simulink library "cex_control_executive_lib"  (R2016b)
settings: Solver=ode45  StartTime=0.0  StopTime=10.0  RelTol=1e-3  EnableMultiTasking=on
undefined symbols (not defined in the file): ase_status_converged, ctl_idle_mode, ctl_stopped_mode, ctl_stopping_mode, ctl_stopping_omega_thresh, ctl_stopping_vel_thresh, tun_ctl_stopped_pos_thresh, tun_ctl_stopped_quat_thresh
libraries: simulink x7, cex_control_executive_lib x1, math_utils x1
settings Model: Creator=jfusco1  LastModifiedBy=jfusco1
settings DataIOCC: LimitDataPoints=on  SaveFormat=Array
settings OptimizationCC: LifeSpan=inf
settings DebuggingCC: AllowSymbolicDim=off  SFUnexpectedBacktrackingDiag=warning  SFNoUnconditionalDefaultTransitionDiag=warning  SFExecutionAtInitializationDiag=none
settings HardwareCC: ProdBitPerPointer=32  ProdBitPerSizeT=32  ProdBitPerPtrDiffT=32  ProdLargestAtomicFloat=None  ProdIntDivRoundTo=Undefined  ProdEndianess=Unspecified  ProdWordSize=32  ProdHWDeviceType=32-bit Generic
settings ModelReferenceCC: PropagateSignalLabelsOutOfModel=off
settings GRTTargetCC: TargetLangStandard=C89/C90 (ANSI)  GeneratePreprocessorConditionals=Disable all
settings ConfigComp: CovMetricSettings=dw  CovHtmlReporting=on  CovSaveCumulativeToWorkspaceVar=on  CovSaveSingleToWorkspaceVar=on  CovExternalEMLEnable=off

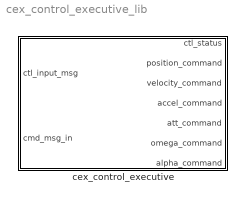
== system cex_control_executive_lib ==
  cex_control_executive : Subsystem

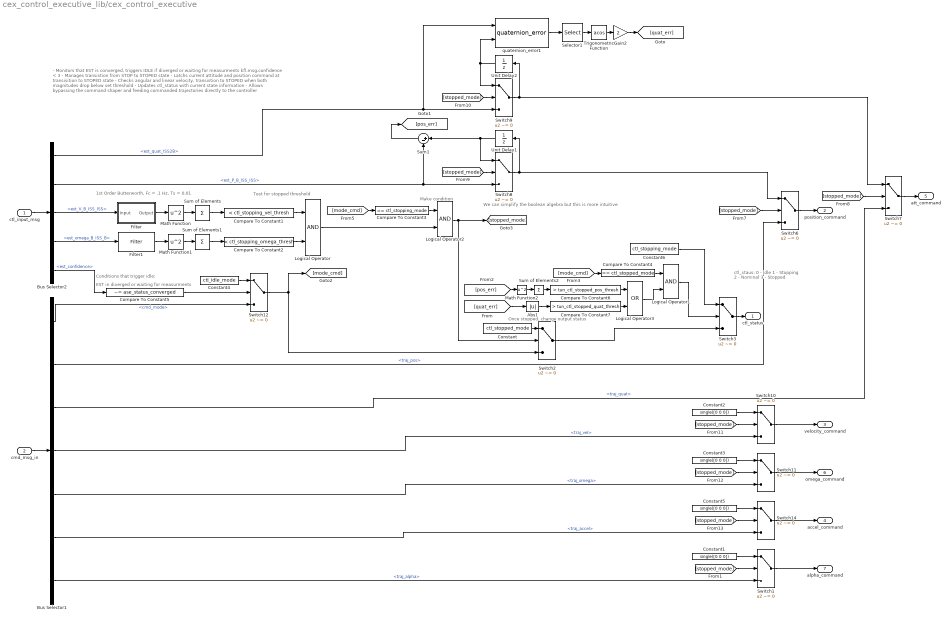
== system cex_control_executive_lib/cex_control_executive ==
  note: ctl_staus:
      | 0 - Idle
      | 1 - Stopping
      | 2 - Nominal
      | 3 - Stopped
  note: 1st Order Butterworth, Fc = .1 Hz, Ts = 0.01
  note: Once stopped, change output status
  note: Make condition
  note: We can simplify the boolean algebra but this is more intuitive
  note: Test for stopped threshold
  note: Conditions that trigger idle:
  note: EST in diverged or waiting for measurments
  note: - Monitors that EST is converged, triggers IDLE if diverged or waiting for measurments kfl.msg.confidence < 3
      | - Manages transistion from STOP to STOPED state
      | 	- Latchs current attitude and position command at transisition to STOPED state
      | 	- Checks angular and linear velocity, transistion to STOPED when both magnitudes drop below set threshold
      | 	- Updates ctl_status with current state information
      | - Allows bypassing the command shaper and feeding commanded trajectories directly to the controller
  ctl_input_msg : Inport  OutDataTypeStr=Bus: ctl_input_msg
  cmd_msg_in : Inport  Port=2  OutDataTypeStr=Bus: cmd_msg
  Abs1 : Abs
  Bus Selector1 : BusSelector  OutputSignals=cmd_mode,traj_pos,traj_quat,traj_vel,traj_omega,traj_accel,traj_alpha
  Bus Selector2 : BusSelector  OutputSignals=est_quat_ISS2B,est_P_B_ISS_ISS,est_V_B_ISS_ISS,est_omega_B_ISS_B,est_confidence
  Compare To Constant1 : simulink/Logic and Bit Operations/Compare To Constant  relop=<  const=ctl_stopping_vel_thresh  OutDataTypeStr=boolean
  Compare To Constant2 : simulink/Logic and Bit Operations/Compare To Constant  relop=<  const=ctl_stopping_omega_thresh  OutDataTypeStr=boolean
  Compare To Constant3 : simulink/Logic and Bit Operations/Compare To Constant  relop===  const=ctl_stopping_mode  OutDataTypeStr=boolean
  Compare To Constant4 : simulink/Logic and Bit Operations/Compare To Constant  relop===  const=ctl_stopped_mode  OutDataTypeStr=boolean
  Compare To Constant5 : simulink/Logic and Bit Operations/Compare To Constant  relop=~=  const=ase_status_converged  OutDataTypeStr=boolean
  Compare To Constant6 : simulink/Logic and Bit Operations/Compare To Constant  relop=>  const=tun_ctl_stopped_pos_thresh  OutDataTypeStr=boolean
  Compare To Constant7 : simulink/Logic and Bit Operations/Compare To Constant  relop=>  const=tun_ctl_stopped_quat_thresh  OutDataTypeStr=boolean
  Constant : Constant  Value=ctl_stopped_mode
  Constant{1..3,5} (4 alike) : Constant  Value=single([0 0 0])
  Constant4 : Constant  Value=ctl_idle_mode
  Constant6 : Constant  Value=ctl_stopping_mode
  Filter : Subsystem  Tag=FilterWizardSubSystem
      settings: ErrorFcn=dspFilterRealizedInBasicElemsAlgLoopErrFcnCallback
  Filter1 : cex_control_executive_lib/cex_control_executive/Filter  Tag=FilterWizardSubSystem
  Gain2 : Gain  Gain=2
  Logical Operator : Logic  AllPortsSameDT=off  OutDataTypeStr=boolean
  Logical Operator1 : Logic  AllPortsSameDT=off  OutDataTypeStr=boolean
  Logical Operator2 : Logic  AllPortsSameDT=off  OutDataTypeStr=boolean
  Logical Operator3 : Logic  Operator=OR  AllPortsSameDT=off  OutDataTypeStr=boolean
  Math Function : Math  Operator=square  SaturateOnIntegerOverflow=on
  Math Function1 : Math  Operator=square  SaturateOnIntegerOverflow=on
  Math Function2 : Math  Operator=square  SaturateOnIntegerOverflow=on
  Selector1 : Selector  InputPortWidth=4  IndexOptions=Index vector (dialog)  Indices=[4]  OutputSizes=1
  Sum of Elements : Sum  Inputs=+
  Sum of Elements1 : Sum  Inputs=+
  Sum of Elements2 : Sum  Inputs=+
  Sum1 : Sum  Inputs=|+-
  Switch{1..3,6..12,14} (11 alike) : Switch  Criteria=u2 ~= 0
  Trigonometric Function : Trigonometry  Operator=acos
  Unit Delay1 : UnitDelay  SampleTime=-1
  Unit Delay2 : UnitDelay  SampleTime=-1
  quaternion_error1 : math_utils/quaternion_error  SystemSampleTime=-1
  ctl_status : Outport
  position_command : Outport  Port=2
  velocity_command : Outport  Port=3
  accel_command : Outport  Port=4
  att_command : Outport  Port=5
  omega_command : Outport  Port=6
  alpha_command : Outport  Port=7
  wires:
  cmd_msg_in/1 -> Bus Selector1/1
  ctl_input_msg/1 -> Bus Selector2/1
  Bus Selector2/3 -> Filter/1(Input)  "<est_V_B_ISS_ISS>"
  Bus Selector2/4 -> Filter1/1  "<est_omega_B_ISS_B>"
  Filter/1(Output) -> Math Function/1
  Math Function/1 -> Sum of Elements/1
  Sum of Elements/1 -> Compare To Constant1/1
  Filter1/1 -> Math Function1/1
  Math Function1/1 -> Sum of Elements1/1
  Sum of Elements1/1 -> Compare To Constant2/1
  Compare To Constant1/1 -> Logical Operator/1
  Compare To Constant2/1 -> Logical Operator/2
  Switch12/1 -> [mode_cmd], Switch2/3
  Constant/1 -> Switch2/1
  Compare To Constant3/1 -> Logical Operator2/1
  Logical Operator2/1 -> [stopped_mode], Switch2/2
  Logical Operator/1 -> Logical Operator2/2
  [mode_cmd] -> Compare To Constant3/1
  [stopped_mode] -> Switch6/2
  [stopped_mode] -> Switch7/2
  Bus Selector1/2 -> Switch6/3  "<traj_pos>"
  Bus Selector1/3 -> Switch7/3  "<traj_quat>"
  Bus Selector1/4 -> Switch10/3  "<traj_vel>"
  Bus Selector1/5 -> Switch11/3  "<traj_omega>"
  Switch8/1 -> Switch6/1, Unit Delay1/1
  Unit Delay1/1 -> Sum1/1, Switch8/1
  Bus Selector2/2 -> Sum1/2, Switch8/3  "<est_P_B_ISS_ISS>"
  [stopped_mode] -> Switch8/2
  Switch9/1 -> Unit Delay2/1, Switch7/1
  Unit Delay2/1 -> quaternion_error1/2, Switch9/1
  [stopped_mode] -> Switch9/2
  Bus Selector2/1 -> quaternion_error1/1, Switch9/3  "<est_quat_ISS2B>"
  Switch6/1 -> position_command/1
  Switch7/1 -> att_command/1
  [stopped_mode] -> Switch10/2
  Switch10/1 -> velocity_command/1
  Constant2/1 -> Switch10/1
  [stopped_mode] -> Switch11/2
  Constant3/1 -> Switch11/1
  Switch11/1 -> omega_command/1
  Bus Selector2/5 -> Compare To Constant5/1  "<est_confidence>"
  Compare To Constant5/1 -> Switch12/2
  Bus Selector1/1 -> Switch12/3  "<cmd_mode>"
  Constant4/1 -> Switch12/1
  Bus Selector1/6 -> Switch14/3  "<traj_accel>"
  [stopped_mode] -> Switch14/2
  Constant5/1 -> Switch14/1
  Switch14/1 -> accel_command/1
  [stopped_mode] -> Switch1/2
  Constant1/1 -> Switch1/1
  Switch1/1 -> alpha_command/1
  Bus Selector1/7 -> Switch1/3  "<traj_alpha>"
  Sum1/1 -> [pos_err]
  Compare To Constant4/1 -> Logical Operator1/1
  [mode_cmd] -> Compare To Constant4/1
  [quat_err] -> Abs1/1
  Abs1/1 -> Compare To Constant7/1
  Selector1/1 -> Trigonometric Function/1
  Trigonometric Function/1 -> Gain2/1
  quaternion_error1/1 -> Selector1/1
  Gain2/1 -> [quat_err]
  Compare To Constant6/1 -> Logical Operator3/1
  Compare To Constant7/1 -> Logical Operator3/2
  Logical Operator3/1 -> Logical Operator1/2
  Switch2/1 -> Switch3/3
  Logical Operator1/1 -> Switch3/2
  Switch3/1 -> ctl_status/1
  Constant6/1 -> Switch3/1
  Math Function2/1 -> Sum of Elements2/1
  Sum of Elements2/1 -> Compare To Constant6/1
  [pos_err] -> Math Function2/1

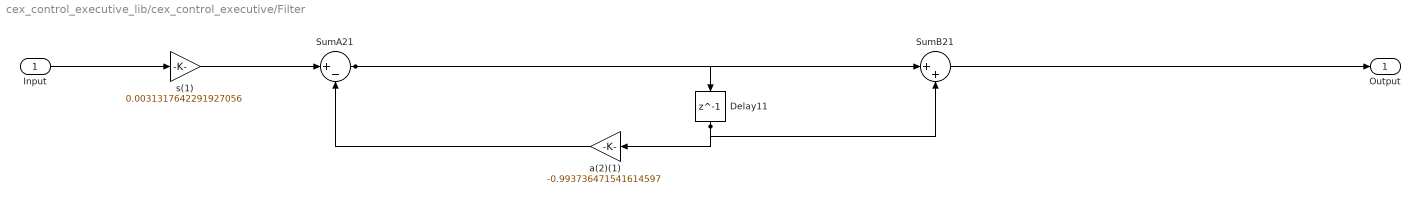
== system cex_control_executive_lib/cex_control_executive/Filter ==
  Input : Inport
  Delay11 : Delay  DelayLength=1  InitialCondition=0
  SumA21 : Sum  Inputs=|+-  RndMeth=Nearest  SaturateOnIntegerOverflow=on  OutDataTypeStr=Inherit: Same as first input
  SumB21 : Sum  Inputs=|++  RndMeth=Nearest  SaturateOnIntegerOverflow=on  OutDataTypeStr=Inherit: Same as first input
  a(2)(1) : Gain  Gain=-0.993736471541614597  ParamDataTypeStr=double  RndMeth=Nearest  SaturateOnIntegerOverflow=on  OutDataTypeStr=Inherit: Same as input
  s(1) : Gain  Gain=0.0031317642291927056  ParamDataTypeStr=double  RndMeth=Nearest  SaturateOnIntegerOverflow=on  OutDataTypeStr=Inherit: Same as input
  Output : Outport
  wires:
  Input/1 -> s(1)/1
  s(1)/1 -> SumA21/1
  SumA21/1 -> SumB21/1, Delay11/1
  SumB21/1 -> Output/1
  a(2)(1)/1 -> SumA21/2
  Delay11/1 -> a(2)(1)/1, SumB21/2
